simulink model "globalMonitor"  (Simulink 8.2)
settings: Solver=ode45  StartTime=0.0  StopTime=inf  RelTol=1e-3
undefined symbols (not defined in the file): DefaultProfile, Take, UserQosProfilesLibrary
libraries: DDSLibrary x4
settings Model: Creator=thomas  LastModifiedBy=thomas
settings DataIOCC: SignalLoggingSaveFormat=Dataset
settings OptimizationCC: ExpressionDepthLimit=128
settings DebuggingCC: FcnCallInpInsideContextMsg=EnableAllAsError  StateNameClashWarn=none
settings GRTTargetCC: CombineOutputUpdateFcns=on  GRTInterface=off

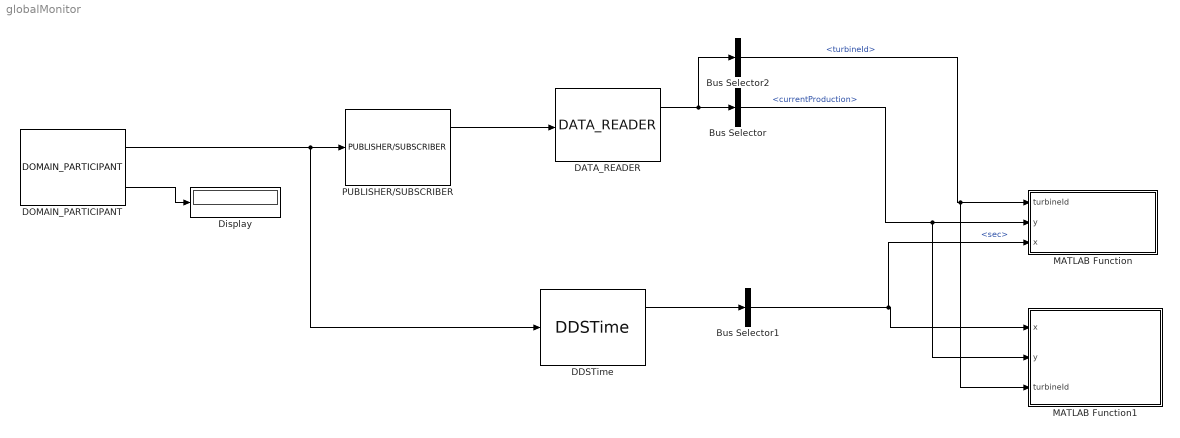
== system globalMonitor ==
  Bus Selector : BusSelector  OutputSignals=currentProduction
  Bus Selector1 : BusSelector  OutputSignals=sec
  Bus Selector2 : BusSelector  OutputSignals=turbineId
  DATA_READER : DDSLibrary/DATA_READER  SFunctionSpec=)  SParam2=Turbine  SParam3=Cluster 1  SParam4=-1  SParam1=on  SParam6=2  SParam7=Take()  SParam5=UserQosProfilesLibrary::DefaultProfile
  DDSTime : DDSLibrary/DDSTime  SFunctionSpec=[]
  DOMAIN_PARTICIPANT : DDSLibrary/DOMAIN_PARTICIPANT  SFunctionSpec=)  SParam1=-1  SParam2=UserQosProfilesLibrary::DefaultProfile  SParam3=0
  Display : Display
  MATLAB Function : MATLAB Function  TreatAsAtomicUnit=on
  MATLAB Function1 : MATLAB Function  TreatAsAtomicUnit=on
  PUBLISHER/SUBSCRIBER : DDSLibrary/PUBLISHER//SUBSCRIBER  SFunctionSpec=)  SParam2=Subscriber  SParam1=-1  SParam3=UserQosProfilesLibrary::DefaultProfile
  wires:
  PUBLISHER/SUBSCRIBER/1 -> DATA_READER/1
  DATA_READER/1 -> Bus Selector2/1, Bus Selector/1
  DOMAIN_PARTICIPANT/2 -> Display/1
  DOMAIN_PARTICIPANT/1 -> DDSTime/1, PUBLISHER/SUBSCRIBER/1
  DDSTime/1 -> Bus Selector1/1
  Bus Selector/1 -> MATLAB Function1/2(y), MATLAB Function/2(y)  "<currentProduction>"
  Bus Selector2/1 -> MATLAB Function1/3(turbineId), MATLAB Function/1(turbineId)  "<turbineId>"
  Bus Selector1/1 -> MATLAB Function/3(x), MATLAB Function1/1(x)  "<sec>"

== matlab function MATLAB Function1 ==
  data: x input double; y input double; turbineId input double
function parkProduction(x, y, turbineId)
% %#codegen
% coder.extrinsic('plot')
% 
% persistent firstRun
% persistent time
% persistent list
% persistent figureHandle
% persistent plotHandle
% 
% s = 100;
% production = 0
% 
% if isempty(firstRun)
%     firstRun = 0
%     time = int32(0)
%     list = zeros([1,s])
%     figureHandle = figure(100)
%     set(figureHandle, 'Name','Simulation Plot Window', 'NumberTitle', 'off')
%     plotHandle = plot(0,0, 'r*')
% end
% 
% if firstRun == 0
%    time = x 
%    firstRun = 1
%    plot(x - time, production, 'r*')
% end
% 
% list(turbineId+1) = y
% 
% for i = 1:s;
%     production = production + list(i)
% end
% 
% figure(figureHandle)
% %plot(x - time, production, 'r*')
% 
% set(plotHandle, 'XData', x - time, 'YData', production)
% 
% hold on

== matlab function MATLAB Function ==
  data: turbineId input double; y input double; x input double
function plotTurbines(turbineId, y, x)
% %#codegen
% 
% persistent firstRun
% persistent time
% persistent figureHandle
% 
% if isempty(firstRun)
%     firstRun = 0
%     time = int32(0)
%     figureHandle = figure(100)
%     set(figureHandle, 'Name','Simulation Plot Window', 'NumberTitle', 'off')
% end
% 
% if firstRun == 0
%    time = x 
%    firstRun = 1
% end
% 
% figure(figureHandle)
% 
% coder.extrinsic('plot')
% plot(x - time, y, '*')
% hold on
% 
% % ih=nsert additional code as needed to turn on grid, setup axis limits,
